simulink model "chap6_6sim"  (Simulink 5.0)
settings: Solver=ode45  StartTime=0.0  StopTime=3  FixedStep=0.001  RelTol=1e-3
settings Model: LastModifiedBy=Administrator  ExtModeTrigMode=oneshot  ExtModeArmWhenConnect=off  LimitDataPoints=off  BooleanDataType=off

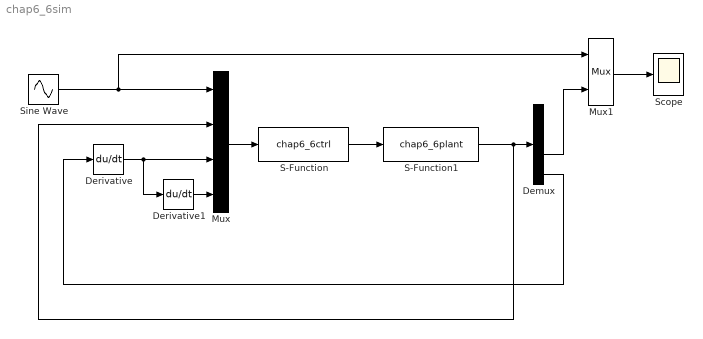
== system chap6_6sim ==
  Demux : Demux
  Derivative : Derivative
  Derivative1 : Derivative
  Mux : Mux
  Mux1 : Mux  Inputs=2
  S-Function : S-Function  FunctionName=chap6_6ctrl
  S-Function1 : S-Function  FunctionName=chap6_6plant
  Scope : Scope
      settings: YMin=-1.1  YMax=1
  Sine Wave : Sin  Frequency=pi  SampleTime=0
  wires:
  Sine Wave/1 -> Mux1/1, Mux/1
  Mux1/1 -> Scope/1
  S-Function/1 -> S-Function1/1
  S-Function1/1 -> Demux/1, Mux/2
  Mux/1 -> S-Function/1
  Demux/3 -> Mux1/2
  Derivative/1 -> Mux/3, Derivative1/1
  Derivative1/1 -> Mux/4
  Demux/4 -> Derivative/1
